simulink model "Product2"  (R2014a)
settings: Solver=FixedStepDiscrete  StartTime=0.0  StopTime=10.0  FixedStep=0.1  RelTol=1e-3
settings Model: CovSFcnEnable=on  BufferReuse=off  Creator=yamasefu  LastModifiedBy=ts1413
settings OptimizationCC: BlockReduction=off  OptimizeBlockIOStorage=off  BufferReuse=off  GlobalBufferReuse=off  ExpressionFolding=off  LocalBlockOutputs=off  OptimizeModelRefInitCode=on  LifeSpan=1  SimCompilerOptimization=off
settings DebuggingCC: MergeDetectMultiDrivingBlocksExec=error  SolverPrmCheckMsg=none  FrameProcessingCompatibilityMsg=error
settings RTWCC: SystemTargetFile=ert.tlc  GenCodeOnly=on  TemplateMakefile=ert_default_tmf  Description=Embedded Coder  RTWCompilerOptimization=off
settings CodeAppCC: IgnoreCustomStorageClasses=off
settings ERTTargetCC: ParMdlRefBuildCompliant=on  CompOptLevelCompliant=on  ConcurrentExecutionCompliant=on  ERTFirstTimeCompliant=on  ModelStepFunctionPrototypeControlCompliant=on  CPPClassGenCompliant=on  InlinedParameterPlacement=Hierarchical  ERTCustomFileTemplate=example_file_process.tlc

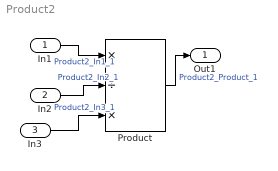
== system Product2 ==
  In1 : Inport
  In2 : Inport  Port=2
  In3 : Inport  Port=3
  Product : Product  Inputs=*/*
  Out1 : Outport
  wires:
  In1/1 -> Product/1  "Product2_In1_1"
  Product/1 -> Out1/1  "Product2_Product_1"
  In2/1 -> Product/2  "Product2_In2_1"
  In3/1 -> Product/3  "Product2_In3_1"
